simulink model "PPS_System"  (R2022b)
settings: configuration reference "PPS_AutosarConfig" (kept outside this file)
libraries: autosarlibdem x1, autosarlibnvm x1, simulink x1
settings Model: DataDictionary=PPS_DD.sldd  Creator=MAAM  LastModifiedBy=MAAM
settings ConfigSetRef: SourceName=PPS_AutosarConfig

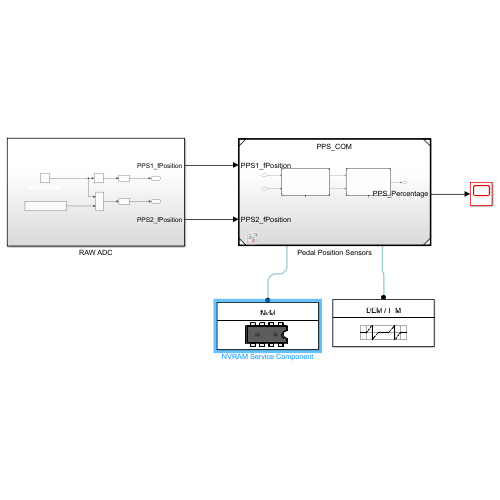
[thumbnail: Simulink's stored preview of the top-level diagram]
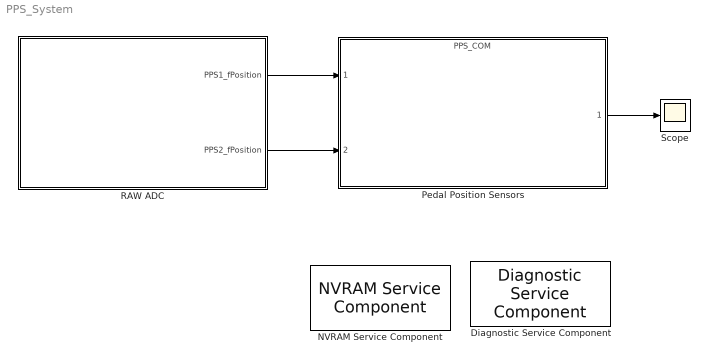
== system PPS_System ==
  Diagnostic Service Component : autosarlibdem/Diagnostic Service Component  ClientPortNames={'PPS1_StuckHigh', 'PPS1_StuckLow', 'PPS2_StuckHigh', 'PPS2_StuckLow', 'PPS_Fail', 'PPS_StuckCoherency'}  ClientPortPortDefinedArguments={'1', '1', '1', '1', '1', '1'}  MaxEventId=10  MaxFID=10  DemDebounceCounterIncrementStepSize=1  DemDebounceCounterDecrementStepSize=1  DemDebounceCounterFailedThreshold=2  DemDebounceCounterPassedThreshold=-1  InhibitionMatrix=zeros(11,'uint8')  EnableConditionIndexes=zeros(257,'uint8')  StorageConditionIndexes=zeros(257,'uint8')
  NVRAM Service Component : autosarlibnvm/NVRAM Service Component  ClientPortNames={'PPS_HighLimit_H_NvMService', 'PPS_HighLimit_L_NvMService', 'PPS_LowLimit_NvMService'}  ClientPortPortDefinedArguments={'135', '136', '235'}  MaxBlockId=10  NvInitValues={'0', '0', '0', '0', '0', '0', '0', '0', '0', '0', '0', '0', '0', '0', '0', '0', '0', '0', '0', '0', '0', '0', '0', '0', '0', '0', '0', '0', '0', '0', '0', '0', '0', '0', '0', '0', '0', '0', '0', '0', '0', '0', '0', '0', '0', '0', '0', '0', '0', '0', '0', '0', '0', '0', '0', '0', '0', '0', '0', '0', '0', '0', '0', '0', '0', '0', '0', '0', '0', '0', '0', '0', '0', '0', '0', '0', '0', '0', '0', '0', '0', '0', '0', '0', '0', '0', '0', '0', '0', '0', '0', '0', '0', '0', '0', '0', '0', '0', '0', '0', '0', '0', '0', '0', '0', '0', '0', '0', '0', '0', '0', '0', '0', '0', '0', '0', '0', '0', '0', '0', '0', '0', '0', '0', '0', '0', '0', '0', '0', '0', '0', '0', '0', '0', '232', '3', '0', '0', '0', '0', '0', '0', '0', '0', '0', '0', '0', '0', '0', '0', '0', '0', '0', '0', '0', '0', '0', '0', '0', '0', '0', '0', '0', '0', '0', '0', '0', '0', '0', '0', '0', '0', '0', '0', '0', '0', '0', '0', '0', '0', '0', '0', '0', '0', '0', '0', '0', '0', '0', '0', '0', '0', '0', '0', '0', '0', '0', '0', '0', '0', '0', '0', '0', '0', '0', '0', '0', '0', '0', '0', '0', '0', '0', '0', '0', '0', '0', '0', '0', '0', '0', '0', '0', '0', '0', '0', '0', '0', '0', '0', '0', '0', '0', '0', '0'}
  Pedal Position Sensors : ModelReference  ModelNameDialog=PPS_COM  SimulationMode=Normal  ModelReferenceVersion=1.4
  RAW ADC : Subsystem
  Scope : Scope
  wires:
  Pedal Position Sensors/1 -> Scope/1
  RAW ADC/1(PPS1_fPosition) -> Pedal Position Sensors/1
  RAW ADC/2(PPS2_fPosition) -> Pedal Position Sensors/2

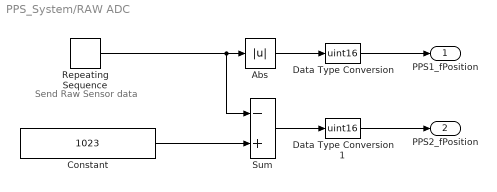
== system PPS_System/RAW ADC ==
  note: Send Raw Sensor data
  Abs : Abs  SaturateOnIntegerOverflow=off
  Constant : Constant  Value=1023  OutDataTypeStr=uint16  SampleTime=-1
  Data Type Conversion : DataTypeConversion  OutDataTypeStr=uint16  SaturateOnIntegerOverflow=off  RndMeth=Floor
  Data Type Conversion1 : DataTypeConversion  OutDataTypeStr=uint16  SaturateOnIntegerOverflow=off  RndMeth=Floor
  Repeating Sequence : simulink/Sources/Repeating Sequence  rep_seq_t=[0 2 4 6 8 10 12 14 16 18 20]  rep_seq_y=[0 500 1200 500 200 1200 -500 1100 0 800 -500]
  Sum : Sum  Inputs=-+  OutDataTypeStr=uint16
  PPS1_fPosition : Outport
  PPS2_fPosition : Outport  Port=2
  wires:
  Abs/1 -> Data Type Conversion/1
  Data Type Conversion1/1 -> PPS2_fPosition/1
  Data Type Conversion/1 -> PPS1_fPosition/1
  Repeating Sequence/1 -> Sum/1, Abs/1
  Constant/1 -> Sum/2
  Sum/1 -> Data Type Conversion1/1
